simulink model "simulink_model"  (R2019b)
settings: Solver=VariableStepAuto  StartTime=0.0  StopTime=10.0  RelTol=1e-3
values from neighbouring files (symbols this model uses):
  K = 51.075    [lab3.m]
  tau = t_rise/2.197    (= 0.021506599909)    [lab3.m]
settings Model: Creator=JasonsRazer  LastModifiedBy=JasonsRazer

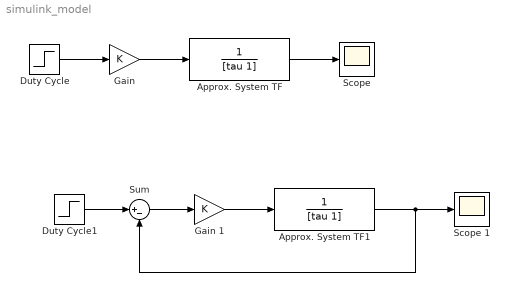
== system simulink_model ==
  Approx. System TF : TransferFcn  Denominator=[tau 1]
  Approx. System TF1 : TransferFcn  Denominator=[tau 1]
  Duty Cycle : Step  Time=0  After=100  SampleTime=0
  Duty Cycle1 : Step  Time=0  After=100  SampleTime=0
  "Gain " : Gain  Gain=K
  Gain 1 : Gain  Gain=K
  "Scope " : Scope
  Scope 1 : Scope
  Sum : Sum  Inputs=|+-
  wires:
  Duty Cycle/1 -> "Gain "/1
  "Gain "/1 -> Approx. System TF/1
  Approx. System TF/1 -> "Scope "/1
  Gain 1/1 -> Approx. System TF1/1
  Approx. System TF1/1 -> Sum/2, Scope 1/1
  Duty Cycle1/1 -> Sum/1
  Sum/1 -> Gain 1/1
